simulink model "untitled"  (R2015a)
settings: Solver=FixedStepDiscrete  StartTime=0.0  StopTime=10.0  FixedStep=1  RelTol=1e-3
settings Model: Creator=sala3  LastModifiedBy=Jesus

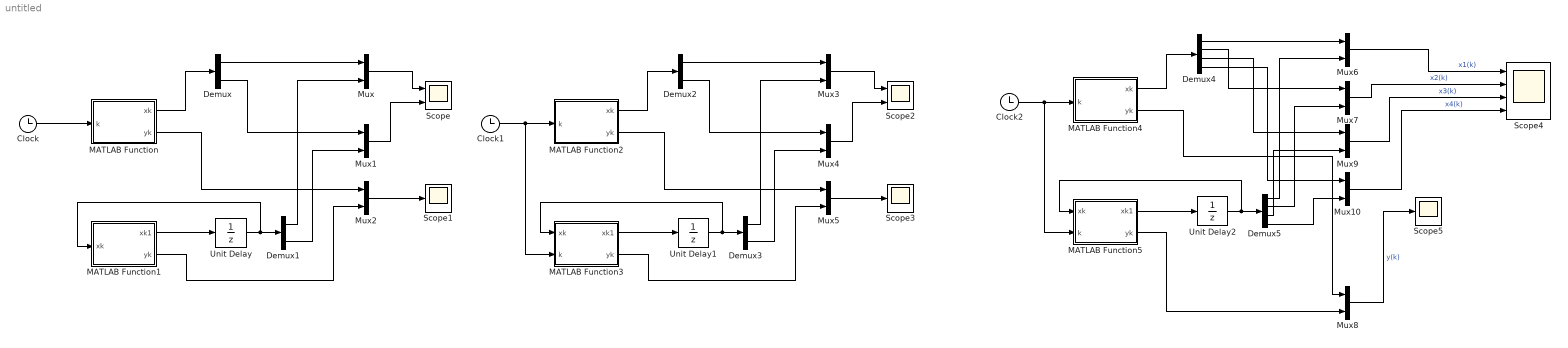
== system untitled ==
  Clock : Clock
  Clock1 : Clock
  Clock2 : Clock
  Demux{,1..3} (4 alike) : Demux  Outputs=2
  Demux4 : Demux
  Demux5 : Demux
  MATLAB Function : MATLAB Function  TreatAsAtomicUnit=on
  MATLAB Function1 : MATLAB Function  TreatAsAtomicUnit=on
  MATLAB Function2 : MATLAB Function  TreatAsAtomicUnit=on
  MATLAB Function3 : MATLAB Function  TreatAsAtomicUnit=on
  MATLAB Function4 : MATLAB Function  TreatAsAtomicUnit=on
  MATLAB Function5 : MATLAB Function  TreatAsAtomicUnit=on
  Mux{,1..10} (11 alike) : Mux  Inputs=2
  Scope : Scope  NumInputPorts=2
      settings: YMin=-5~-5  YMax=5~5
  Scope1 : Scope
  Scope2 : Scope  NumInputPorts=2
      settings: YMin=-5~-5  YMax=5~5  SaveName=ScopeData2
  Scope3 : Scope
      settings: SaveName=ScopeData3
  Scope4 : Scope  NumInputPorts=4
      settings: YMin=-5~-5~-5~-5  YMax=5~5~5~5  SaveName=ScopeData4
  Scope5 : Scope
      settings: SaveName=ScopeData5
  Unit Delay : UnitDelay  InitialCondition=[2 -2]  SampleTime=-1
  Unit Delay1 : UnitDelay  InitialCondition=[2 -2]  SampleTime=-1
  Unit Delay2 : UnitDelay  InitialCondition=[-1 1 -2 2]  SampleTime=-1
  wires:
  Clock/1 -> MATLAB Function/1(k)
  MATLAB Function/1(xk) -> Demux/1
  MATLAB Function1/1(xk1) -> Unit Delay/1
  Unit Delay/1 -> Demux1/1, MATLAB Function1/1(xk)
  Mux/1 -> Scope/1
  Demux/1 -> Mux/1
  Demux1/1 -> Mux/2
  Mux1/1 -> Scope/2
  Demux/2 -> Mux1/1
  Demux1/2 -> Mux1/2
  MATLAB Function1/2(yk) -> Mux2/2
  Mux2/1 -> Scope1/1
  MATLAB Function/2(yk) -> Mux2/1
  Clock1/1 -> MATLAB Function3/2(k), MATLAB Function2/1(k)
  MATLAB Function2/1(xk) -> Demux2/1
  MATLAB Function3/1(xk1) -> Unit Delay1/1
  Unit Delay1/1 -> MATLAB Function3/1(xk), Demux3/1
  Mux3/1 -> Scope2/1
  Demux2/1 -> Mux3/1
  Demux3/1 -> Mux3/2
  Mux4/1 -> Scope2/2
  Demux2/2 -> Mux4/1
  Demux3/2 -> Mux4/2
  MATLAB Function3/2(yk) -> Mux5/2
  Mux5/1 -> Scope3/1
  MATLAB Function2/2(yk) -> Mux5/1
  Clock2/1 -> MATLAB Function4/1(k), MATLAB Function5/2(k)
  MATLAB Function4/1(xk) -> Demux4/1
  MATLAB Function5/1(xk1) -> Unit Delay2/1
  Unit Delay2/1 -> Demux5/1, MATLAB Function5/1(xk)
  Mux6/1 -> Scope4/1  "x1(k)"
  Demux4/1 -> Mux6/1
  Demux5/1 -> Mux6/2
  Mux7/1 -> Scope4/2  "x2(k)"
  Demux4/2 -> Mux7/1
  Demux5/2 -> Mux7/2
  MATLAB Function5/2(yk) -> Mux8/2
  Mux8/1 -> Scope5/1  "y(k)"
  MATLAB Function4/2(yk) -> Mux8/1
  Mux9/1 -> Scope4/3  "x3(k)"
  Mux10/1 -> Scope4/4  "x4(k)"
  Demux4/3 -> Mux9/1
  Demux4/4 -> Mux10/1
  Demux5/3 -> Mux9/2
  Demux5/4 -> Mux10/2

== matlab function untitled/MATLAB Function1 ==
  data: xk1 output; xk input; yk output
function [xk1,yk] = fcn(xk)
%#codegen
A=[2 .5;0 .8];
B=[-5;2];
C=[1 -1];
u=1;
xk1=A*xk+B*u;
yk=C*xk;

== matlab function untitled/MATLAB Function ==
  data: xk output; k input; yk output
function [xk,yk] = fcn(k)
%#codegen
 xk=[5*(4/5)^k - 3*2^k;10 - 12*(4/5)^k];
 yk=17*(4/5)^k - 3*2^k - 10;

== matlab function untitled/MATLAB Function2 ==
  data: xk output; k input; yk output
function [xk,yk] = fcn(k)
%#codegen
 xk=[ 5*k - 3*2^k + 5*(4/5)^k;10 - 12*(4/5)^k];
 yk=5*k - 3*2^k + 17*(4/5)^k - 10;

== matlab function untitled/MATLAB Function3 ==
  data: xk1 output; xk input; yk output; k input
function [xk1,yk] = fcn(xk,k)
%#codegen
A=[2 .5;0 .8];
B=[0,-5;2,0];
C=[1 -1];
u=[1;k];
xk1=A*xk+B*u;
yk=C*xk;

== matlab function untitled/MATLAB Function4 ==
  data: xk output; k input; yk output
function [xk,yk] = fcn(k)
%#codegen
 xk=[-(233*(-2)^k)/144-2^k/16-(19*(-2)^k*(k-1))/24-1/9;(19*(-2)^k)/12 - 2^k/4 - 1/3 ;- 2^k - 1;(7*(-3)^k)/4 + 1/4];
 yk=(7*(-3)^k)/4 - 2^k - 3/4;

== matlab function untitled/MATLAB Function5 ==
  data: xk1 output; xk input; yk output; k input
function [xk1,yk] = fcn(xk,k)
%#codegen
A=[-2 1 0 0;0 -2 1 0;0 0 2 0;0 0 0 -3];
B=[0 0 1 1]';
C=[0 0 1 1];
u=1;
xk1=A*xk+B*u;
yk=C*xk;
